simulink library "tp333079"  (Simulink 5.0)
values from neighbouring files (symbols this model uses):
  b = 1    [main_flock3.m]    (also in main_flock4.m; params_flocking_ros.m)
undefined symbols (not defined in the file or in its folder): AC, AlphaBnd, BetaBnd, CDda, CDde, CDdf, CDdr, CDM, CDmin, CGempty, CGgross, CL0, CLa, CLalphadot, Clbeta, Clda, CLde, CLdf, Cldr, CLM, CLmind, Clp, CLq, Clr, Cm0, Cma, Cmalphadot, Cmde, Cmdf, CmM, Cmq, Cnbeta, Cnda, Cndr, Cnp, Cnr, CP, CT, CYbeta, CYda, CYdr, CYp, CYr, Displacement, dmy, Engine, EulerIni, FuelFlow, FuelIni, J, Jempty, Jeng, Jgross, Jprop, MAC, MAP, MAPLim, MassIni, MaxPower, mempty ... (+26)
libraries: aerosimlib x325, simulink3 x42
(part 3 of 11)

== system tp333079/Atmosphere/Wind Shear ==
  note: Transversal wind shear
  note: Time derivatives of wind speed
      | in body axes
  note: Body velocities
  note: Lateral wind shear
  note: Vertical wind shear
  WindAcc : Inport  Port=1  PortDimensions=[3 1]  SampleTime=-1  DataType=auto
      settings: SignalType=auto
  TurbAcc : Inport  Port=2  PortDimensions=[3 1]  SampleTime=-1  DataType=auto
      settings: SignalType=auto
  Velocities : Inport  Port=3  PortDimensions=[3 1]  SampleTime=-1  DataType=auto
      settings: SignalType=auto
  Demux : Demux  Outputs=3  BusSelectionMode=off
  Demux1 : Demux  Outputs=3  BusSelectionMode=off
  Derivative : Derivative
  Mux : Mux  Inputs=3
  Mux1 : Mux  Inputs=3
  Product1 : Product  Inputs=*/  Multiplication=Element-wise(.*)  SaturateOnIntegerOverflow=on
  Product2 : Product  Inputs=*/  Multiplication=Element-wise(.*)  SaturateOnIntegerOverflow=on
  Product3 : Product  Inputs=*/  Multiplication=Element-wise(.*)  SaturateOnIntegerOverflow=on
  Sum : Sum  Inputs=|++  SaturateOnIntegerOverflow=on
  Terminator : Terminator
  Terminator1 : Terminator
  Terminator2 : Terminator
  Zero : Constant  Value=0
  Zero Offset : aerosimlib/Math/Zero Offset  tol=10^-6
  Zero Offset1 : Subsystem  SimViewingDevice=off  mask(Zero offset){tol=10^-6}
      mask prompts: tol "Tolerance"
      mask help: This block outputs a value equal to the tolerance specified in the block parameters if the input falls within a sphere with this tolerance as radius and center in the origin. Otherwise, the output equals the input.
      settings: Permissions=ReadWrite  RTWFcnNameOpts=Auto  RTWFileNameOpts=Auto
  Zero Offset2 : Subsystem  SimViewingDevice=off  mask(Zero offset){tol=10^-6}
      mask prompts: tol "Tolerance"
      mask help: This block outputs a value equal to the tolerance specified in the block parameters if the input falls within a sphere with this tolerance as radius and center in the origin. Otherwise, the output equals the input.
      settings: Permissions=ReadWrite  RTWFcnNameOpts=Auto  RTWFileNameOpts=Auto
  WindAngRates : Outport  Port=1
  WindAngAcc : Outport  Port=2
  wires:
  Product3/1 -> Terminator2/1
  Mux1/1 -> Derivative/1
  Zero Offset2/1(Out) -> Product1/2
  Zero Offset1/1(Out) -> Product2/2
  Derivative/1 -> WindAngAcc/1
  Sum/1 -> Demux1/1
  TurbAcc/1 -> Sum/2
  WindAcc/1 -> Sum/1
  Mux/1 -> WindAngRates/1
  Zero/1 -> Mux/1, Mux1/1, Mux1/3, Mux1/2
  Demux1/2 -> Product2/1
  Demux1/3 -> Product1/1, Product3/1
  Demux1/1 -> Terminator/1
  Velocities/1 -> Demux/1
  Demux/1 -> Zero Offset2/1(In), Zero Offset1/1(In)
  Demux/2 -> Zero Offset/1
  Demux/3 -> Terminator1/1
  Product1/1 -> Mux/2
  Product2/1 -> Mux/3
  Zero Offset/1 -> Product3/2

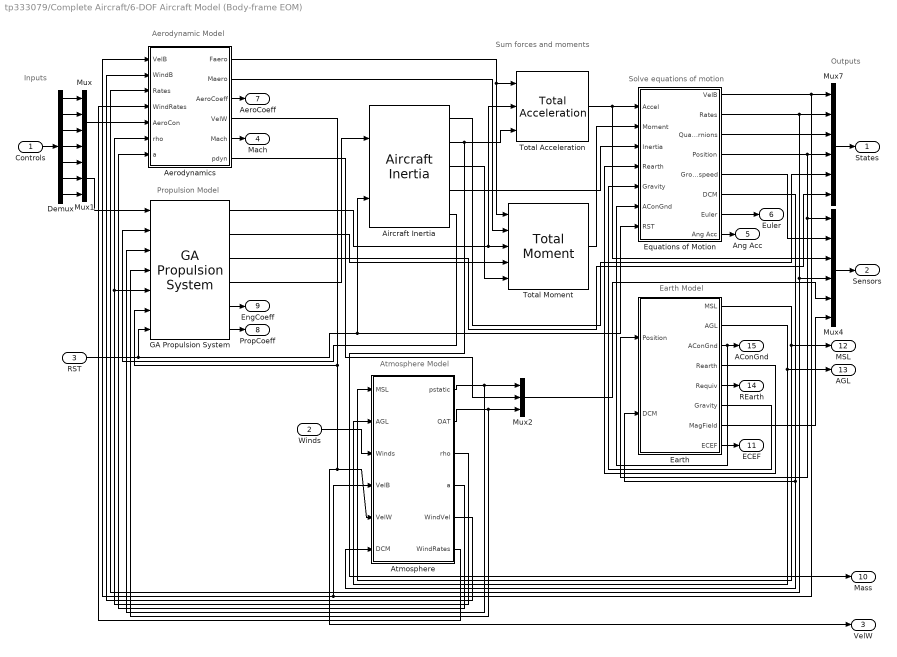
== system tp333079/Complete Aircraft/6-DOF Aircraft Model (Body-frame EOM) ==
  note: Propulsion Model
  note: Atmosphere Model
  note: Sum forces and moments
  note: Earth Model
  note: Aerodynamic Model
  note: Outputs
  note: Inputs
  note: Solve equations of motion
  Controls : Inport  Port=1  PortDimensions=-1  SampleTime=-1  DataType=auto
      settings: SignalType=auto
  Winds : Inport  Port=2  PortDimensions=-1  SampleTime=-1  DataType=auto
      settings: SignalType=auto
  RST : Inport  Port=3  PortDimensions=-1  SampleTime=-1  DataType=auto
      settings: SignalType=auto
  Aerodynamics : Subsystem  SimViewingDevice=off
      settings: Permissions=ReadWrite  RTWFcnNameOpts=Auto  RTWFileNameOpts=Auto
  Aircraft Inertia : aerosimlib/Inertia/Aircraft Inertia  FuelIni=FuelIni  Mempty=mempty  Mgross=mgross  CGempty=CGempty  CGgross=CGgross  Jempty=Jempty  Jgross=Jgross
  Atmosphere : Subsystem  SimViewingDevice=off
      settings: Permissions=ReadWrite  RTWFcnNameOpts=Auto  RTWFileNameOpts=Auto
  Demux : Demux  Outputs=7  BusSelectionMode=off
  Earth : Subsystem  SimViewingDevice=off
      settings: Permissions=ReadWrite  RTWFcnNameOpts=Auto  RTWFileNameOpts=Auto
  Equations of Motion : Subsystem  SimViewingDevice=off
      settings: Permissions=ReadWrite  RTWFcnNameOpts=Auto  RTWFileNameOpts=Auto
  GA Propulsion System : aerosimlib/Propulsion/GA Propulsion System  OmegaIni=OmegaIni  RPM=RPM  MAP=MAP  FuelFlow=FuelFlow  Power=Power  Jeng=Jeng  J=J  CT=CT  CP=CP  Rprop=Rprop  Jprop=Jprop  TSL=TSL
  Mux : Mux  Inputs=4
  Mux1 : Mux  Inputs=3
  Mux2 : Mux  Inputs=3
  Mux4 : Mux  Inputs=6
  Mux7 : Mux  Inputs=6
  Total Acceleration : aerosimlib/Equations of Motion/Total Acceleration
  Total Moment : aerosimlib/Equations of Motion/Total Moment  raero=rAC  rprop=rHub
  States : Outport  Port=1
  Sensors : Outport  Port=2
  VelW : Outport  Port=3
  Mach : Outport  Port=4
  Ang Acc : Outport  Port=5
  Euler : Outport  Port=6
  AeroCoeff : Outport  Port=7
  PropCoeff : Outport  Port=8
  EngCoeff : Outport  Port=9
  Mass : Outport  Port=10
  ECEF : Outport  Port=11
  MSL : Outport  Port=12
  AGL : Outport  Port=13
  REarth : Outport  Port=14
  AConGnd : Outport  Port=15
  wires:
  Earth/8(ECEF) -> ECEF/1
  Aerodynamics/3(AeroCoeff) -> AeroCoeff/1
  Aerodynamics/5(Mach) -> Mach/1
  Equations of Motion/3(Quaternions) -> Mux7/3
  Mux/1 -> Aerodynamics/5(AeroCon)
  Equations of Motion/4(Position) -> Mux7/4, Mux4/1, Earth/1(Position)
  Equations of Motion/2(Rates) -> Mux7/2, Mux4/4, Aerodynamics/3(Rates)
  Equations of Motion/1(VelB) -> Mux7/1, Atmosphere/4(VelB), Aerodynamics/1(VelB)
  Mux1/1 -> GA Propulsion System/1
  Mux7/1 -> States/1
  Mux4/1 -> Sensors/1
  Controls/1 -> Demux/1
  Demux/1 -> Mux/1
  Demux/2 -> Mux/2
  Demux/3 -> Mux/3
  Demux/4 -> Mux/4
  Demux/5 -> Mux1/1
  Demux/6 -> Mux1/2
  Demux/7 -> Mux1/3
  GA Propulsion System/5 -> EngCoeff/1
  GA Propulsion System/6 -> PropCoeff/1
  Earth/5(Requiv) -> REarth/1
  Earth/3(AConGnd) -> AConGnd/1, Equations of Motion/6(AConGnd)
  Equations of Motion/5(Groundspeed) -> Mux4/2
  Total Acceleration/1 -> Equations of Motion/1(Accel), Mux4/3
  Earth/7(MagField) -> Mux4/6
  Earth/6(Gravity) -> Equations of Motion/5(Gravity)
  Earth/4(Rearth) -> Equations of Motion/4(Rearth)
  Aircraft Inertia/2 -> Total Acceleration/3, Mass/1
  Aircraft Inertia/4 -> Equations of Motion/3(Inertia)
  Total Moment/1 -> Equations of Motion/2(Moment)
  Aircraft Inertia/3 -> Total Moment/5
  Aerodynamics/1(Faero) -> Total Acceleration/1, Total Moment/1
  Aerodynamics/2(Maero) -> Total Moment/2
  GA Propulsion System/1 -> Total Acceleration/2, Total Moment/3
  GA Propulsion System/2 -> Total Moment/4
  Equations of Motion/6(DCM) -> Earth/2(DCM), Atmosphere/6(DCM)
  Atmosphere/1(pstatic) -> Mux2/1, GA Propulsion System/3
  Atmosphere/2(OAT) -> Mux2/3, GA Propulsion System/4
  Aerodynamics/6(pdyn) -> Mux2/2
  Mux2/1 -> Mux4/5
  Aircraft Inertia/1 -> Mux7/5
  GA Propulsion System/3 -> Mux7/6
  GA Propulsion System/4 -> Aircraft Inertia/1
  Aerodynamics/4(VelW) -> GA Propulsion System/6, Atmosphere/5(VelW), VelW/1
  Earth/1(MSL) -> Atmosphere/1(MSL), MSL/1
  Earth/2(AGL) -> Atmosphere/2(AGL), AGL/1
  Winds/1 -> Atmosphere/3(Winds)
  Atmosphere/5(WindVel) -> Aerodynamics/2(WindB)
  Atmosphere/3(rho) -> Aerodynamics/6(rho), GA Propulsion System/5
  Atmosphere/4(a) -> Aerodynamics/7(a)
  Aircraft Inertia/5 -> GA Propulsion System/2
  RST/1 -> GA Propulsion System/7, Equations of Motion/7(RST), Aircraft Inertia/2
  Atmosphere/6(WindRates) -> Aerodynamics/4(WindRates)
  Equations of Motion/8(Ang Acc) -> Ang Acc/1
  Equations of Motion/7(Euler) -> Euler/1

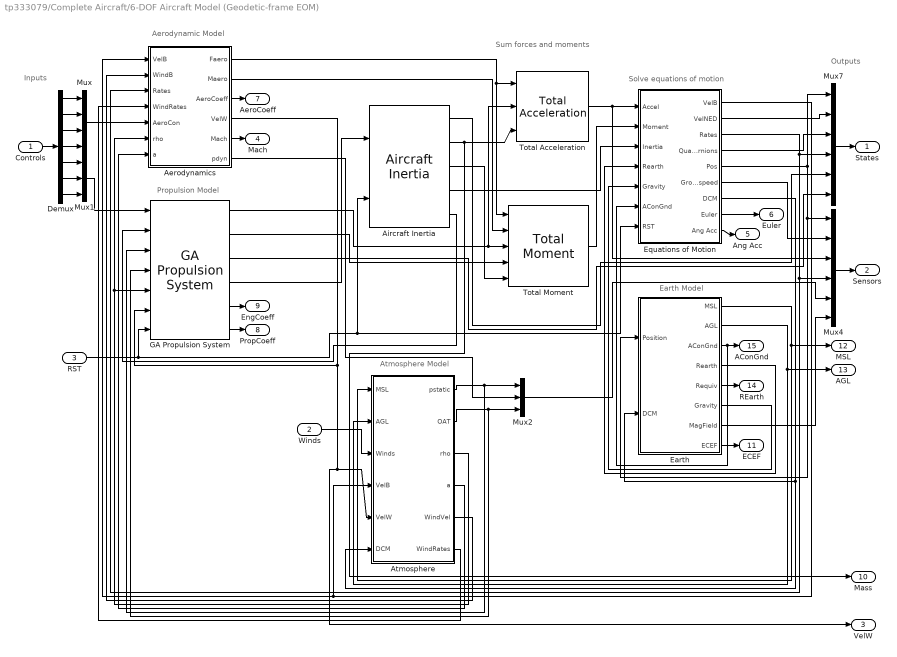
== system tp333079/Complete Aircraft/6-DOF Aircraft Model (Geodetic-frame EOM) ==
  note: Propulsion Model
  note: Atmosphere Model
  note: Sum forces and moments
  note: Earth Model
  note: Aerodynamic Model
  note: Outputs
  note: Inputs
  note: Solve equations of motion
  Controls : Inport  Port=1  PortDimensions=-1  SampleTime=-1  DataType=auto
      settings: SignalType=auto
  Winds : Inport  Port=2  PortDimensions=-1  SampleTime=-1  DataType=auto
      settings: SignalType=auto
  RST : Inport  Port=3  PortDimensions=-1  SampleTime=-1  DataType=auto
      settings: SignalType=auto
  Aerodynamics : Subsystem  SimViewingDevice=off
      settings: Permissions=ReadWrite  RTWFcnNameOpts=Auto  RTWFileNameOpts=Auto
  Aircraft Inertia : aerosimlib/Inertia/Aircraft Inertia  FuelIni=FuelIni  Mempty=mempty  Mgross=mgross  CGempty=CGempty  CGgross=CGgross  Jempty=Jempty  Jgross=Jgross
  Atmosphere : Subsystem  SimViewingDevice=off
      settings: Permissions=ReadWrite  RTWFcnNameOpts=Auto  RTWFileNameOpts=Auto
  Demux : Demux  Outputs=7  BusSelectionMode=off
  Earth : Subsystem  SimViewingDevice=off
      settings: Permissions=ReadWrite  RTWFcnNameOpts=Auto  RTWFileNameOpts=Auto
  Equations of Motion : Subsystem  SimViewingDevice=off
      settings: Permissions=ReadWrite  RTWFcnNameOpts=Auto  RTWFileNameOpts=Auto
  GA Propulsion System : aerosimlib/Propulsion/GA Propulsion System  OmegaIni=OmegaIni  RPM=RPM  MAP=MAP  FuelFlow=FuelFlow  Power=Power  Jeng=Jeng  J=J  CT=CT  CP=CP  Rprop=Rprop  Jprop=Jprop  TSL=TSL
  Mux : Mux  Inputs=4
  Mux1 : Mux  Inputs=3
  Mux2 : Mux  Inputs=3
  Mux4 : Mux  Inputs=6
  Mux7 : Mux  Inputs=6
  Total Acceleration : aerosimlib/Equations of Motion/Total Acceleration
  Total Moment : aerosimlib/Equations of Motion/Total Moment  raero=rAC  rprop=rHub
  States : Outport  Port=1
  Sensors : Outport  Port=2
  VelW : Outport  Port=3
  Mach : Outport  Port=4
  Ang Acc : Outport  Port=5
  Euler : Outport  Port=6
  AeroCoeff : Outport  Port=7
  PropCoeff : Outport  Port=8
  EngCoeff : Outport  Port=9
  Mass : Outport  Port=10
  ECEF : Outport  Port=11
  MSL : Outport  Port=12
  AGL : Outport  Port=13
  REarth : Outport  Port=14
  AConGnd : Outport  Port=15
  wires:
  Earth/8(ECEF) -> ECEF/1
  Aerodynamics/3(AeroCoeff) -> AeroCoeff/1
  Aerodynamics/5(Mach) -> Mach/1
  Mux/1 -> Aerodynamics/5(AeroCon)
  Equations of Motion/5(Pos) -> Mux4/1, Earth/1(Position), Mux7/1
  Equations of Motion/3(Rates) -> Mux4/4, Aerodynamics/3(Rates), Mux7/4
  Equations of Motion/1(VelB) -> Atmosphere/4(VelB), Aerodynamics/1(VelB)
  Mux1/1 -> GA Propulsion System/1
  Mux7/1 -> States/1
  Mux4/1 -> Sensors/1
  Controls/1 -> Demux/1
  Demux/1 -> Mux/1
  Demux/2 -> Mux/2
  Demux/3 -> Mux/3
  Demux/4 -> Mux/4
  Demux/5 -> Mux1/1
  Demux/6 -> Mux1/2
  Demux/7 -> Mux1/3
  GA Propulsion System/5 -> EngCoeff/1
  GA Propulsion System/6 -> PropCoeff/1
  Earth/5(Requiv) -> REarth/1
  Earth/3(AConGnd) -> AConGnd/1, Equations of Motion/6(AConGnd)
  Equations of Motion/6(Groundspeed) -> Mux4/2
  Total Acceleration/1 -> Equations of Motion/1(Accel), Mux4/3
  Earth/7(MagField) -> Mux4/6
  Earth/6(Gravity) -> Equations of Motion/5(Gravity)
  Earth/4(Rearth) -> Equations of Motion/4(Rearth)
  Aircraft Inertia/2 -> Total Acceleration/3, Mass/1
  Aircraft Inertia/4 -> Equations of Motion/3(Inertia)
  Total Moment/1 -> Equations of Motion/2(Moment)
  Aircraft Inertia/3 -> Total Moment/5
  Aerodynamics/1(Faero) -> Total Acceleration/1, Total Moment/1
  Aerodynamics/2(Maero) -> Total Moment/2
  GA Propulsion System/1 -> Total Acceleration/2, Total Moment/3
  GA Propulsion System/2 -> Total Moment/4
  Equations of Motion/7(DCM) -> Earth/2(DCM), Atmosphere/6(DCM)
  Atmosphere/1(pstatic) -> Mux2/1, GA Propulsion System/3
  Atmosphere/2(OAT) -> Mux2/3, GA Propulsion System/4
  Aerodynamics/6(pdyn) -> Mux2/2
  Mux2/1 -> Mux4/5
  Aircraft Inertia/1 -> Mux7/5
  GA Propulsion System/3 -> Mux7/6
  GA Propulsion System/4 -> Aircraft Inertia/1
  Aerodynamics/4(VelW) -> GA Propulsion System/6, Atmosphere/5(VelW), VelW/1
  Earth/1(MSL) -> Atmosphere/1(MSL), MSL/1
  Earth/2(AGL) -> Atmosphere/2(AGL), AGL/1
  Winds/1 -> Atmosphere/3(Winds)
  Atmosphere/5(WindVel) -> Aerodynamics/2(WindB)
  Atmosphere/3(rho) -> Aerodynamics/6(rho), GA Propulsion System/5
  Atmosphere/4(a) -> Aerodynamics/7(a)
  Aircraft Inertia/5 -> GA Propulsion System/2
  RST/1 -> GA Propulsion System/7, Equations of Motion/7(RST), Aircraft Inertia/2
  Atmosphere/6(WindRates) -> Aerodynamics/4(WindRates)
  Equations of Motion/9(Ang Acc) -> Ang Acc/1
  Equations of Motion/8(Euler) -> Euler/1
  Equations of Motion/2(VelNED) -> Mux7/2
  Equations of Motion/4(Quaternions) -> Mux7/3

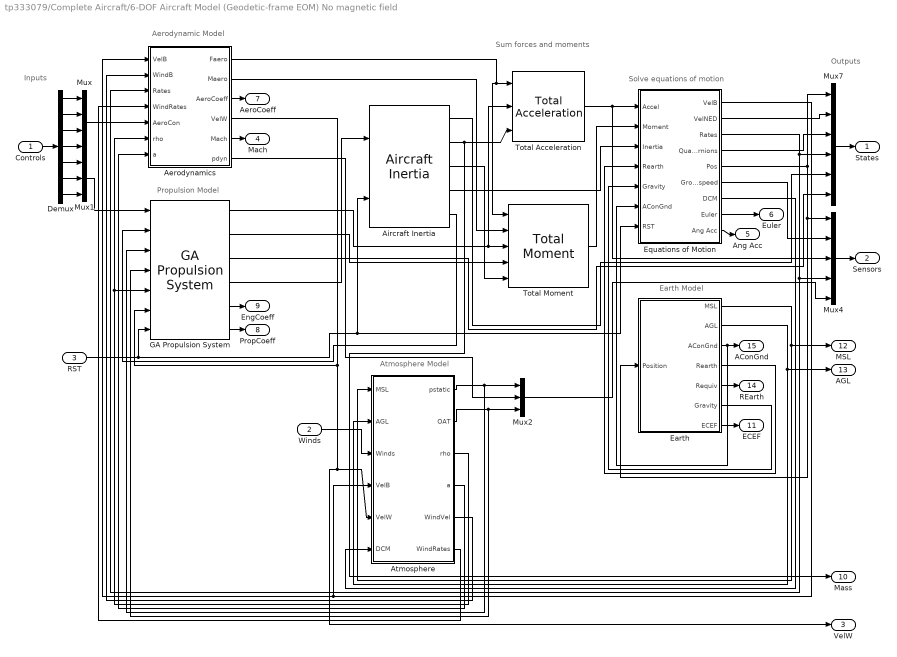
== system tp333079/Complete Aircraft/6-DOF Aircraft Model (Geodetic-frame EOM) No magnetic field ==
  note: Solve equations of motion
  note: Inputs
  note: Outputs
  note: Aerodynamic Model
  note: Earth Model
  note: Sum forces and moments
  note: Atmosphere Model
  note: Propulsion Model
  Controls : Inport  Port=1  PortDimensions=-1  SampleTime=-1  DataType=auto
      settings: SignalType=auto
  Winds : Inport  Port=2  PortDimensions=-1  SampleTime=-1  DataType=auto
      settings: SignalType=auto
  RST : Inport  Port=3  PortDimensions=-1  SampleTime=-1  DataType=auto
      settings: SignalType=auto
  Aerodynamics : Subsystem  SimViewingDevice=off
      settings: Permissions=ReadWrite  RTWFcnNameOpts=Auto  RTWFileNameOpts=Auto
  Aircraft Inertia : aerosimlib/Inertia/Aircraft Inertia  FuelIni=FuelIni  Mempty=mempty  Mgross=mgross  CGempty=CGempty  CGgross=CGgross  Jempty=Jempty  Jgross=Jgross
  Atmosphere : Subsystem  SimViewingDevice=off
      settings: Permissions=ReadWrite  RTWFcnNameOpts=Auto  RTWFileNameOpts=Auto
  Demux : Demux  Outputs=7  BusSelectionMode=off
  Earth : Subsystem  SimViewingDevice=off
      settings: Permissions=ReadWrite  RTWFcnNameOpts=Auto  RTWFileNameOpts=Auto
  Equations of Motion : Subsystem  SimViewingDevice=off
      settings: Permissions=ReadWrite  RTWFcnNameOpts=Auto  RTWFileNameOpts=Auto
  GA Propulsion System : aerosimlib/Propulsion/GA Propulsion System  OmegaIni=OmegaIni  RPM=RPM  MAP=MAP  FuelFlow=FuelFlow  Power=Power  Jeng=Jeng  J=J  CT=CT  CP=CP  Rprop=Rprop  Jprop=Jprop  TSL=TSL
  Mux : Mux  Inputs=4
  Mux1 : Mux  Inputs=3
  Mux2 : Mux  Inputs=3
  Mux4 : Mux  Inputs=5
  Mux7 : Mux  Inputs=6
  Total Acceleration : aerosimlib/Equations of Motion/Total Acceleration
  Total Moment : aerosimlib/Equations of Motion/Total Moment  raero=rAC  rprop=rHub
  States : Outport  Port=1
  Sensors : Outport  Port=2
  VelW : Outport  Port=3
  Mach : Outport  Port=4
  Ang Acc : Outport  Port=5
  Euler : Outport  Port=6
  AeroCoeff : Outport  Port=7
  PropCoeff : Outport  Port=8
  EngCoeff : Outport  Port=9
  Mass : Outport  Port=10
  ECEF : Outport  Port=11
  MSL : Outport  Port=12
  AGL : Outport  Port=13
  REarth : Outport  Port=14
  AConGnd : Outport  Port=15
  wires:
  Equations of Motion/4(Quaternions) -> Mux7/3
  Equations of Motion/2(VelNED) -> Mux7/2
  Equations of Motion/8(Euler) -> Euler/1
  Equations of Motion/9(Ang Acc) -> Ang Acc/1
  Atmosphere/6(WindRates) -> Aerodynamics/4(WindRates)
  RST/1 -> Aircraft Inertia/2, Equations of Motion/7(RST), GA Propulsion System/7
  Aircraft Inertia/5 -> GA Propulsion System/2
  Atmosphere/4(a) -> Aerodynamics/7(a)
  Atmosphere/3(rho) -> GA Propulsion System/5, Aerodynamics/6(rho)
  Atmosphere/5(WindVel) -> Aerodynamics/2(WindB)
  Winds/1 -> Atmosphere/3(Winds)
  Earth/2(AGL) -> AGL/1, Atmosphere/2(AGL)
  Earth/1(MSL) -> MSL/1, Atmosphere/1(MSL)
  Aerodynamics/4(VelW) -> VelW/1, Atmosphere/5(VelW), GA Propulsion System/6
  GA Propulsion System/4 -> Aircraft Inertia/1
  GA Propulsion System/3 -> Mux7/6
  Aircraft Inertia/1 -> Mux7/5
  Mux2/1 -> Mux4/5
  Aerodynamics/6(pdyn) -> Mux2/2
  Atmosphere/2(OAT) -> GA Propulsion System/4, Mux2/3
  Atmosphere/1(pstatic) -> GA Propulsion System/3, Mux2/1
  Equations of Motion/7(DCM) -> Atmosphere/6(DCM)
  GA Propulsion System/2 -> Total Moment/4
  GA Propulsion System/1 -> Total Acceleration/2, Total Moment/3
  Aerodynamics/1(Faero) -> Total Acceleration/1, Total Moment/1
  Aircraft Inertia/3 -> Total Moment/5
  Total Moment/1 -> Equations of Motion/2(Moment)
  Aircraft Inertia/4 -> Equations of Motion/3(Inertia)
  Aircraft Inertia/2 -> Total Acceleration/3, Mass/1
  Earth/4(Rearth) -> Equations of Motion/4(Rearth)
  Earth/6(Gravity) -> Equations of Motion/5(Gravity)
  Total Acceleration/1 -> Mux4/3, Equations of Motion/1(Accel)
  Equations of Motion/6(Groundspeed) -> Mux4/2
  Earth/3(AConGnd) -> Equations of Motion/6(AConGnd), AConGnd/1
  Earth/5(Requiv) -> REarth/1
  GA Propulsion System/6 -> PropCoeff/1
  GA Propulsion System/5 -> EngCoeff/1
  Demux/7 -> Mux1/3
  Demux/6 -> Mux1/2
  Demux/5 -> Mux1/1
  Demux/4 -> Mux/4
  Demux/3 -> Mux/3
  Demux/2 -> Mux/2
  Demux/1 -> Mux/1
  Controls/1 -> Demux/1
  Mux4/1 -> Sensors/1
  Mux7/1 -> States/1
  Mux1/1 -> GA Propulsion System/1
  Equations of Motion/1(VelB) -> Aerodynamics/1(VelB), Atmosphere/4(VelB)
  Equations of Motion/3(Rates) -> Mux7/4, Mux4/4, Aerodynamics/3(Rates)
  Equations of Motion/5(Pos) -> Mux7/1, Earth/1(Position), Mux4/1
  Mux/1 -> Aerodynamics/5(AeroCon)
  Aerodynamics/5(Mach) -> Mach/1
  Aerodynamics/3(AeroCoeff) -> AeroCoeff/1
  Earth/7(ECEF) -> ECEF/1
  Aerodynamics/2(Maero) -> Total Moment/2

== system tp333079/Complete Aircraft/Glider Model ==
  note: Sum forces and moments
  note: Aerodynamic Model
  note: Outputs
  note: Inputs
  note: Solve equations of motion
  Controls : Inport  Port=1  PortDimensions=-1  SampleTime=-1  DataType=auto
      settings: SignalType=auto
  Aerodynamics : aerosimlib/Complete Aircraft/6-DOF Aircraft Model (Body-frame EOM)/Aerodynamics  SimViewingDevice=off
      settings: Permissions=ReadWrite  RTWFcnNameOpts=Auto  RTWFileNameOpts=Auto
  Aircraft Inertia : aerosimlib/Inertia/Aircraft Inertia  FuelIni=0  Mempty=mempty  Mgross=mgross  CGempty=CGempty  CGgross=CGgross  Jempty=Jempty  Jgross=Jgross
  Constant{,5,7..8} (4 alike) : Constant  Value=0
  Constant3 : Constant  Value=zeros(3,1)
  Constant4 : Constant  Value=zeros(3,1)
  Demux1 : Demux  Outputs=3  BusSelectionMode=off
  Equations of Motion : Subsystem  SimViewingDevice=off
      settings: Permissions=ReadWrite  RTWFcnNameOpts=Auto  RTWFileNameOpts=Auto
  Mux2 : Mux  Inputs=3
  Mux3 : Mux  Orientation=left  Inputs=2
  Mux4 : Mux  Inputs=5
  Mux7 : Mux  Inputs=4
  Standard Atmosphere : aerosimlib/Atmosphere/Standard Atmosphere
  Terminator{1..6} (6 alike) : Terminator
  Total Acceleration : aerosimlib/Equations of Motion/Total Acceleration
  Total Moment : aerosimlib/Equations of Motion/Total Moment  raero=rAC  rprop=rHub
  WGS-84 : aerosimlib/Earth/WGS-84  Orientation=left
  States : Outport  Port=1
  Sensors : Outport  Port=2
  VelW : Outport  Port=3
  Mach : Outport  Port=4
  Ang Acc : Outport  Port=5
  Euler : Outport  Port=6
  AeroCoeff : Outport  Port=7
  wires:
  Aerodynamics/3 -> AeroCoeff/1
  Aerodynamics/5 -> Mach/1
  Equations of Motion/3(Quaternions) -> Mux7/3
  Equations of Motion/4(Position) -> Mux7/4, Mux4/1, Demux1/1, WGS-84/1
  Equations of Motion/2(Rates) -> Mux7/2, Mux4/4, Aerodynamics/3
  Equations of Motion/1(VelB) -> Mux7/1, Aerodynamics/1
  Mux7/1 -> States/1
  Mux4/1 -> Sensors/1
  Controls/1 -> Aerodynamics/5
  Equations of Motion/5(Groundspeed) -> Mux4/2
  Total Acceleration/1 -> Equations of Motion/1(Accel), Mux4/3
  Aircraft Inertia/2 -> Total Acceleration/3
  Aircraft Inertia/4 -> Equations of Motion/3(Inertia)
  Total Moment/1 -> Equations of Motion/2(Moment)
  Aircraft Inertia/3 -> Total Moment/5
  Aerodynamics/1 -> Total Acceleration/1, Total Moment/1
  Aerodynamics/2 -> Total Moment/2
  Aerodynamics/6 -> Mux2/2
  Mux2/1 -> Mux4/5
  Aerodynamics/4 -> VelW/1
  Equations of Motion/7(Euler) -> Euler/1
  Equations of Motion/8(Ang Acc) -> Ang Acc/1
  Constant/1 -> Equations of Motion/6(AConGnd)
  Constant7/1 -> Equations of Motion/7(RST)
  Equations of Motion/6(DCM) -> Terminator2/1
  Demux1/1 -> Terminator1/1
  Demux1/2 -> Terminator3/1
  Demux1/3 -> Standard Atmosphere/1
  Standard Atmosphere/1 -> Mux2/1
  Standard Atmosphere/2 -> Mux2/3
  Standard Atmosphere/3 -> Aerodynamics/6
  Standard Atmosphere/4 -> Aerodynamics/7
  Constant3/1 -> Aerodynamics/2
  Constant4/1 -> Aerodynamics/4
  Constant8/1 -> Aircraft Inertia/2
  Constant5/1 -> Aircraft Inertia/1
  Aircraft Inertia/5 -> Terminator4/1
  Aircraft Inertia/1 -> Terminator5/1
  WGS-84/1 -> Mux3/1
  WGS-84/2 -> Mux3/2
  WGS-84/3 -> Terminator6/1
  Mux3/1 -> Equations of Motion/4(Rearth)
  WGS-84/4 -> Equations of Motion/5(Gravity)

== system tp333079/Complete Aircraft/Inertial Navigation System ==
  IMU : Inport  Port=1  PortDimensions=[6 1]  SampleTime=tsamp  DataType=auto
      settings: SignalType=auto
  RST : Inport  Port=2  PortDimensions=1  SampleTime=tsamp  DataType=auto
      settings: SignalType=auto
  Attitude : aerosimlib/Equations of Motion/Body-Frame EOM/Kinematics (Quaternions)  QuaternionsIni=QuaternionsIni
  Body-Inertial DCM : aerosimlib/Transformations/Body-Inertial DCM From Quaternions  Orientation=left
  Constant : Constant  Value=0
  Demux : Demux  Outputs=2  BusSelectionMode=off
  Mux : Mux  Inputs=3
  Position : aerosimlib/Equations of Motion/Geodetic-Frame EOM/Position  PositionIni=PositionIni
  Terminator : Terminator
  Velocity : aerosimlib/Equations of Motion/Geodetic-Frame EOM/Velocity  VelocitiesIni=VelocitiesIni
  WGS-84 : aerosimlib/Earth/WGS-84
  PVA : Outport  Port=1
  wires:
  IMU/1 -> Demux/1
  WGS-84/3 -> Terminator/1
  Velocity/1 -> Position/1, Mux/2
  WGS-84/1 -> Position/2
  WGS-84/2 -> Position/3
  WGS-84/4 -> Velocity/5
  Demux/1 -> Velocity/3
  Demux/2 -> Attitude/1
  RST/1 -> Attitude/2, Position/5, Velocity/6
  Attitude/1 -> Mux/3, Body-Inertial DCM/1
  Position/1 -> Velocity/1, WGS-84/1, Mux/1
  Position/2 -> Velocity/2
  Constant/1 -> Position/4
  Mux/1 -> PVA/1
  Body-Inertial DCM/1 -> Velocity/4

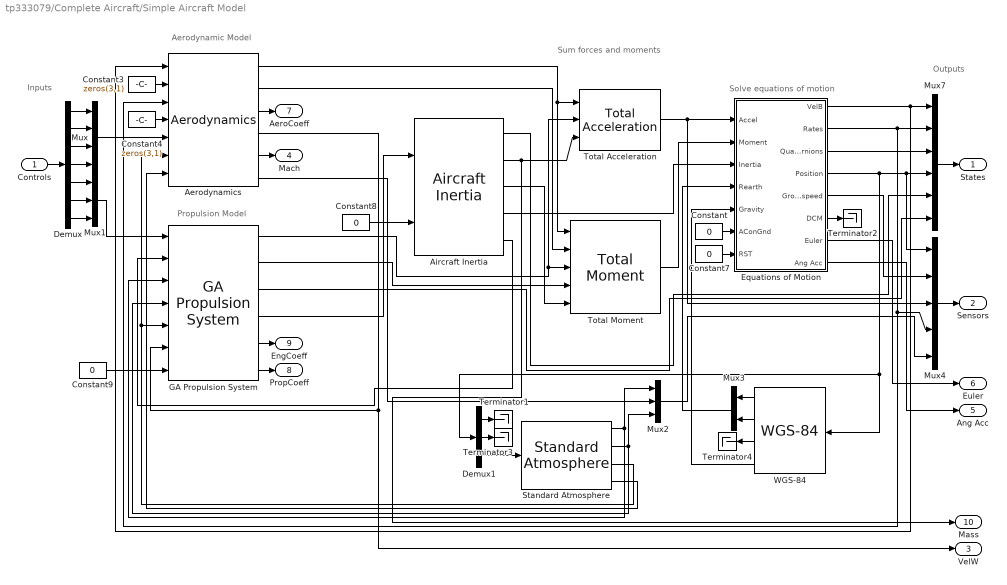
== system tp333079/Complete Aircraft/Simple Aircraft Model ==
  note: Propulsion Model
  note: Sum forces and moments
  note: Aerodynamic Model
  note: Outputs
  note: Inputs
  note: Solve equations of motion
  Controls : Inport  Port=1  PortDimensions=-1  SampleTime=-1  DataType=auto
      settings: SignalType=auto
  Aerodynamics : aerosimlib/Complete Aircraft/6-DOF Aircraft Model (Body-frame EOM)/Aerodynamics  SimViewingDevice=off
      settings: Permissions=ReadWrite  RTWFcnNameOpts=Auto  RTWFileNameOpts=Auto
  Aircraft Inertia : aerosimlib/Inertia/Aircraft Inertia  FuelIni=FuelIni  Mempty=mempty  Mgross=mgross  CGempty=CGempty  CGgross=CGgross  Jempty=Jempty  Jgross=Jgross
  Constant{,7..9} (4 alike) : Constant  Value=0
  Constant3 : Constant  Value=zeros(3,1)
  Constant4 : Constant  Value=zeros(3,1)
  Demux : Demux  Outputs=7  BusSelectionMode=off
  Demux1 : Demux  Outputs=3  BusSelectionMode=off
  Equations of Motion : Subsystem  SimViewingDevice=off
      settings: Permissions=ReadWrite  RTWFcnNameOpts=Auto  RTWFileNameOpts=Auto
  GA Propulsion System : aerosimlib/Propulsion/GA Propulsion System  OmegaIni=OmegaIni  RPM=RPM  MAP=MAP  FuelFlow=FuelFlow  Power=Power  Jeng=Jeng  J=J  CT=CT  CP=CP  Rprop=Rprop  Jprop=Jprop  TSL=TSL
  Mux : Mux  Inputs=4
  Mux1 : Mux  Inputs=3
  Mux2 : Mux  Inputs=3
  Mux3 : Mux  Orientation=left  Inputs=2
  Mux4 : Mux  Inputs=5
  Mux7 : Mux  Inputs=6
  Standard Atmosphere : aerosimlib/Atmosphere/Standard Atmosphere
  Terminator{1..4} (4 alike) : Terminator
  Total Acceleration : aerosimlib/Equations of Motion/Total Acceleration
  Total Moment : aerosimlib/Equations of Motion/Total Moment  raero=rAC  rprop=rHub
  WGS-84 : aerosimlib/Earth/WGS-84  Orientation=left
  States : Outport  Port=1
  Sensors : Outport  Port=2
  VelW : Outport  Port=3
  Mach : Outport  Port=4
  Ang Acc : Outport  Port=5
  Euler : Outport  Port=6
  AeroCoeff : Outport  Port=7
  PropCoeff : Outport  Port=8
  EngCoeff : Outport  Port=9
  Mass : Outport  Port=10
  wires:
  Aerodynamics/3 -> AeroCoeff/1
  Aerodynamics/5 -> Mach/1
  Equations of Motion/3(Quaternions) -> Mux7/3
  Mux/1 -> Aerodynamics/5
  Equations of Motion/4(Position) -> Mux7/4, Mux4/1, Demux1/1, WGS-84/1
  Equations of Motion/2(Rates) -> Mux7/2, Mux4/4, Aerodynamics/3
  Equations of Motion/1(VelB) -> Mux7/1, Aerodynamics/1
  Mux1/1 -> GA Propulsion System/1
  Mux7/1 -> States/1
  Mux4/1 -> Sensors/1
  Controls/1 -> Demux/1
  Demux/1 -> Mux/1
  Demux/2 -> Mux/2
  Demux/3 -> Mux/3
  Demux/4 -> Mux/4
  Demux/5 -> Mux1/1
  Demux/6 -> Mux1/2
  Demux/7 -> Mux1/3
  GA Propulsion System/5 -> EngCoeff/1
  GA Propulsion System/6 -> PropCoeff/1
  Equations of Motion/5(Groundspeed) -> Mux4/2
  Total Acceleration/1 -> Equations of Motion/1(Accel), Mux4/3
  Aircraft Inertia/2 -> Mass/1, Total Acceleration/3
  Aircraft Inertia/4 -> Equations of Motion/3(Inertia)
  Total Moment/1 -> Equations of Motion/2(Moment)
  Aircraft Inertia/3 -> Total Moment/5
  Aerodynamics/1 -> Total Acceleration/1, Total Moment/1
  GA Propulsion System/1 -> Total Acceleration/2, Total Moment/3
  GA Propulsion System/2 -> Total Moment/4
  Aerodynamics/6 -> Mux2/2
  Mux2/1 -> Mux4/5
  Aircraft Inertia/1 -> Mux7/5
  GA Propulsion System/3 -> Mux7/6
  GA Propulsion System/4 -> Aircraft Inertia/1
  Aerodynamics/4 -> GA Propulsion System/6, VelW/1
  Aircraft Inertia/5 -> GA Propulsion System/2
  Equations of Motion/7(Euler) -> Euler/1
  Equations of Motion/8(Ang Acc) -> Ang Acc/1
  Constant/1 -> Equations of Motion/6(AConGnd)
  Constant7/1 -> Equations of Motion/7(RST)
  Equations of Motion/6(DCM) -> Terminator2/1
  Demux1/1 -> Terminator1/1
  Demux1/2 -> Terminator3/1
  Demux1/3 -> Standard Atmosphere/1
  Standard Atmosphere/1 -> Mux2/1, GA Propulsion System/3
  Standard Atmosphere/2 -> Mux2/3, GA Propulsion System/4
  Standard Atmosphere/3 -> Aerodynamics/6, GA Propulsion System/5
  Standard Atmosphere/4 -> Aerodynamics/7
  Constant3/1 -> Aerodynamics/2
  Constant4/1 -> Aerodynamics/4
  Constant8/1 -> Aircraft Inertia/2
  Constant9/1 -> GA Propulsion System/7
  Aerodynamics/2 -> Total Moment/2
  WGS-84/1 -> Mux3/1
  WGS-84/2 -> Mux3/2
  Mux3/1 -> Equations of Motion/4(Rearth)
  WGS-84/4 -> Equations of Motion/5(Gravity)
  WGS-84/3 -> Terminator4/1

== system tp333079/Earth/EGM-96 ==
  note: Sources
  note: Compute Mean-Sea Level Altitude
  Position : Inport  Port=1  PortDimensions=-1  SampleTime=-1  DataType=auto
      settings: SignalType=auto
  Demux2 : Demux  Outputs=3  BusSelectionMode=off
  Longitude Bound 0-2pi : Subsystem  SimViewingDevice=off
      settings: Permissions=ReadWrite  RTWFcnNameOpts=Auto  RTWFileNameOpts=Auto
      mask Type: Longitude bound
      mask Description: Bounds the longitude to [0, 2pi]. When 0 bound is exceeded the longitude wraps back to 2pi; when the 2pi bound is exceeded the longitude wraps back to 0.
  Look-Up Table (2-D) : simulink3/Functions & Tables/Look-Up Table (2-D)  x=Lat  y=Lon  t=Alterr'
  Sum : Sum  Inputs=+++  SaturateOnIntegerOverflow=on
  WGS-84 correction : Constant  Value=-0.53
  rad 2 deg : Subsystem  SimViewingDevice=off
      settings: Permissions=ReadWrite  RTWFcnNameOpts=Auto  RTWFileNameOpts=Auto
      mask Type: Radians to degrees
      mask Description: Convert radians to degrees.
      mask Display: disp('RAD DEG');
  rad 2 deg1 : Subsystem  SimViewingDevice=off
      settings: Permissions=ReadWrite  RTWFcnNameOpts=Auto  RTWFileNameOpts=Auto
      mask Type: Radians to degrees
      mask Description: Convert radians to degrees.
      mask Display: disp('RAD DEG');
  MSLAlt : Outport  Port=1
  wires:
  Longitude Bound 0-2pi/1(Out) -> rad 2 deg1/1(In)
  Position/1 -> Demux2/1
  Demux2/3 -> Sum/1
  Demux2/1 -> rad 2 deg/1(In)
  Demux2/2 -> Longitude Bound 0-2pi/1(In)
  rad 2 deg/1(Out) -> Look-Up Table (2-D)/1
  rad 2 deg1/1(Out) -> Look-Up Table (2-D)/2
  Look-Up Table (2-D)/1 -> Sum/2
  WGS-84 correction/1 -> Sum/3
  Sum/1 -> MSLAlt/1

== system tp333079/Earth/Ground Detection ==
  MSLAlt : Inport  Port=1  PortDimensions=-1  SampleTime=-1  DataType=auto
      settings: SignalType=auto
  GndAlt : Inport  Port=2  PortDimensions=-1  SampleTime=-1  DataType=auto
      settings: SignalType=auto
  False : Constant  Value=0
  Sum : Sum  Inputs=|+-  SaturateOnIntegerOverflow=on
  Switch : Switch  Threshold=0
  True : Constant  Value=1
  AConGnd : Outport  Port=1
  AGLAlt : Outport  Port=2
  wires:
  MSLAlt/1 -> Sum/1
  GndAlt/1 -> Sum/2
  Sum/1 -> Switch/2, AGLAlt/1
  False/1 -> Switch/1
  True/1 -> Switch/3
  Switch/1 -> AConGnd/1

== system tp333079/Earth/WGS-84 ==
  note: Sources
  note: Compute radii and surface gravity
  note: Correct gravity for altitude
  note: Outputs
  Position : Inport  Port=1  PortDimensions=-1  SampleTime=-1  DataType=auto
      settings: SignalType=auto
  1/2 : Constant  Value=1/2
  3/2 : Constant  Value=3/2
  Demux2 : Demux  Outputs=3  BusSelectionMode=off
  Equatorial Radius : Constant  Value=6378137
  First Eccentricity : Constant  Value=0.0818191908426
  Gravity at Equator : Constant  Value=9.7803267714
  Gravity formula const : Constant  Value=0.00193185138639
  Math Function : Math  Operator=pow  OutputSignalType=auto
  Math Function1 : Math  Operator=pow  OutputSignalType=auto
  Mux : Mux  Inputs=3
  One : Constant  Value=1
  Product : Product  Inputs=2  Multiplication=Element-wise(.*)  SaturateOnIntegerOverflow=on
  Product1 : Product  Inputs=**/  Multiplication=Element-wise(.*)  SaturateOnIntegerOverflow=on
  Product2 : Product  Inputs=*/  Multiplication=Element-wise(.*)  SaturateOnIntegerOverflow=on
  Product3 : Product  Inputs=2  Multiplication=Element-wise(.*)  SaturateOnIntegerOverflow=on
  Product4 : Product  Inputs=**/  Multiplication=Element-wise(.*)  SaturateOnIntegerOverflow=on
  Product5 : Product  Inputs=2  Multiplication=Element-wise(.*)  SaturateOnIntegerOverflow=on
  Sum : Sum  Inputs=|+-  SaturateOnIntegerOverflow=on
  Sum1 : Sum  Inputs=|+-  SaturateOnIntegerOverflow=on
  Sum2 : Sum  Inputs=|++  SaturateOnIntegerOverflow=on
  Terminator : Terminator
  eps^2 : Math  Operator=square  OutputSignalType=auto
  g(phi,h) : Fcn  Expr=u[1]-(3.0877e-6 - 0.0044e-6*u[2])*u[3]+0.072e-12*u[3]*u[3]
  sin(phi) : Trigonometry  Operator=sin  OutputSignalType=auto
  sin(phi)^2 : Math  Operator=square  OutputSignalType=auto
  sqrt : Math  Operator=sqrt  OutputSignalType=auto
  Rmeridian : Outport  Port=1
  Rnormal : Outport  Port=2
  Re : Outport  Port=3
  Gravity : Outport  Port=4
  wires:
  sqrt/1 -> Re/1
  Product5/1 -> sqrt/1
  First Eccentricity/1 -> eps^2/1
  eps^2/1 -> Sum/2, Product/1
  sin(phi)/1 -> sin(phi)^2/1
  sin(phi)^2/1 -> Product/2, Product3/2, Mux/2
  One/1 -> Sum1/1, Sum2/1, Sum/1
  Product/1 -> Sum1/2
  Sum1/1 -> Math Function/1, Math Function1/1
  3/2/1 -> Math Function/2
  1/2/1 -> Math Function1/2
  Equatorial Radius/1 -> Product1/1, Product2/1
  Sum/1 -> Product1/2
  Math Function/1 -> Product1/3
  Math Function1/1 -> Product2/2, Product4/3
  Product1/1 -> Rmeridian/1, Product5/1
  Product2/1 -> Rnormal/1, Product5/2
  Gravity formula const/1 -> Product3/1
  Product3/1 -> Sum2/2
  Gravity at Equator/1 -> Product4/1
  Sum2/1 -> Product4/2
  Product4/1 -> Mux/1
  Position/1 -> Demux2/1
  Demux2/1 -> sin(phi)/1
  Demux2/2 -> Terminator/1
  Mux/1 -> g(phi,h)/1
  g(phi,h)/1 -> Gravity/1
  Demux2/3 -> Mux/3

== system tp333079/Earth/WMM-2000 ==
  Position : Inport  Port=1  PortDimensions=[3 1]  SampleTime=-1  DataType=double
      settings: SignalType=auto
  DCM : Inport  Port=2  PortDimensions=[3 3]  SampleTime=-1  DataType=double
      settings: SignalType=auto
  Date : Constant  Value=simdate
  DayToYear : Gain  Gain=1/365  Multiplication=Element-wise(K.*u)  SaturateOnIntegerOverflow=on
  Demux : Demux  Outputs=3  BusSelectionMode=off
  Demux1 : Demux  Outputs=3  BusSelectionMode=off
  MonthToYear : Gain  Gain=1/12  Multiplication=Element-wise(K.*u)  SaturateOnIntegerOverflow=on
  Mux : Mux  Inputs=3
  Product : Product  Inputs=2  Multiplication=Matrix(*)  SaturateOnIntegerOverflow=on
  S-Function : S-Function  FunctionName=sfunwmm  Parameters=wmmfile  PortCounts=[]  SFunctionModules=''
  Sum : Sum  Inputs=+++  SaturateOnIntegerOverflow=on
  MagField : Outport  Port=1
  wires:
  S-Function/1 -> Product/2
  DCM/1 -> Product/1
  Date/1 -> Demux/1
  Demux/1 -> DayToYear/1
  DayToYear/1 -> Sum/1
  Demux/2 -> MonthToYear/1
  Demux/3 -> Sum/3
  MonthToYear/1 -> Sum/2
  Position/1 -> S-Function/1
  Sum/1 -> S-Function/2
  Product/1 -> Demux1/1
  Demux1/1 -> Mux/1
  Demux1/2 -> Mux/2
  Demux1/3 -> Mux/3
  Mux/1 -> MagField/1

== system tp333079/Equations of Motion/Body-Frame EOM ==
  Forces : Subsystem  SimViewingDevice=off  mask(Force equations){VelocitiesIni=VelocitiesIni}
      mask prompts: VelocitiesIni "Initial velocities:"
      mask help: 6-DOF rigid body force equations.
      settings: Permissions=ReadWrite  RTWFcnNameOpts=Auto  RTWFileNameOpts=Auto
      mask Help:
      | The block implements the 6-DOF rigid-body force equations.
      | <P><B>Inputs:</B>
      | <LI>Rates = the 3x1 vector of body angular rates</LI>
      | <LI>Accel = the 3x1 vector of linear body accelerations</LI>
      | <LI>Gravity = the gravitational acceleration at current location.
      | <LI>DCM = the 3x3 rotation matrix from navigation to body frame.
      | <LI>RST = the integrator reset flag (rising edge)</LI>
      | </P>
      | <P><B>Output:</B>
      | <LI>Velocities = the 3x1 vector of aircraft velocities in body axes</LI>
      | </P>
      | <P><B>Parameters:</B>
      | <LI>Initial velocities = the 3x1 vector of initial aircraft velocities</LI>
      | </P>
  Kinematics (Euler) : Subsystem  SimViewingDevice=off  mask(Kinematic Equations){EulerIni=EulerIni}
      mask prompts: EulerIni "Initial Euler angles:"
      mask help: 6-DOF rigid body kinematic equations, using Euler angles.
      settings: Permissions=ReadWrite  RTWFcnNameOpts=Auto  RTWFileNameOpts=Auto
      mask Help:
      | The block implements the 6-DOF rigid-body kinematic equations, using Euler angles.
      | <P><B>Inputs:</B>
      | <LI>Rates = the 3x1 vector of body angular rates</LI>
      | <LI>RST = the integrator reset flag (rising edge)</LI>
      | </P>
      | <P><B>Output:</B>
      | <LI>Euler = the 3x1 vector of Euler angles</LI>
      | </P>
      | <P><B>Parameters:</B>
      | <LI>Initial Euler angles = the 3x1 vector of initial body attitude</LI>
      | </P>
  Kinematics (Quaternions) : Subsystem  SimViewingDevice=off  mask(Kinematic Equations){QuaternionsIni=QuaternionsIni}
      mask prompts: QuaternionsIni "Initial quaternions:"
      mask help: 6-DOF rigid body kinematic equations, using Euler-Rodrigues quaternions.
      settings: Permissions=ReadWrite  RTWFcnNameOpts=Auto  RTWFileNameOpts=Auto
      mask Help:
      | The block implements the 6-DOF rigid-body kinematic equations, using Euler-Rodrigues quaternions.
      | <P><B>Inputs:</B>
      | <LI>Rates = the 3x1 vector of body angular rates</LI>
      | <LI>RST = the integrator reset flag (rising edge)</LI>
      | </P>
      | <P><B>Output:</B>
      | <LI>Quaternions = the 4x1 vector of body quaternions</LI>
      | </P>
      | <P><B>Parameters:</B>
      | <LI>Initial quaternions = the 4x1 vector of initial body quaternions</LI>
      | </P>
  Moments : Subsystem  SimViewingDevice=off  mask(Moment equations){RatesIni=RatesIni}
      mask prompts: RatesIni "Initial angular rates:"
      mask help: 6-DOF rigid body moment equations.
      settings: Permissions=ReadWrite  RTWFcnNameOpts=Auto  RTWFileNameOpts=Auto
      mask Help:
      | The block implements the 6-DOF rigid-body moment equations.
      | <P><B>Inputs:</B>
      | <LI>Inertia = the 10x1 vector of inertia coefficients</LI>
      | <LI>Moments = the 3x1 vector of airframe moments</LI>
      | <LI>RST = the integrator reset flag (rising edge)</LI>
      | </P>
      | <P><B>Output:</B>
      | <LI>Angular Rates = the 3x1 vector of body angular rates</LI>
      | <LI>Angular Acc = the 3x1 vector of body angular accelerations.
      | </P>
      | <P><B>Parameters:</B>
      | <LI>Initial rates = the 3x1 vector of initial angular rates</LI>
      | </P>
  Navigation : Subsystem  SimViewingDevice=off  mask(Navigation equations){PositionIni=PositionIni}
      mask prompts: PositionIni "Initial position:"
      mask help: 6-DOF rigid body navigation equations.
      settings: Permissions=ReadWrite  RTWFcnNameOpts=Auto  RTWFileNameOpts=Auto
      mask Help:
      | The block implements the inertial navigation equations.
      | <P><B>Inputs:</B>
      | <LI>Velocities = the 3x1 vector of aircraft velocities in body axes</LI>
      | <LI>DCM = the 3x3 frame transformation from navigation frame to body frame</LI>
      | <LI>Rmeridian = the Earth meridian radius, in m</LI>
      | <LI>Rnormal = the Earth normal radius, in m</LI>
      | <LI>AConGnd = the aircraft-on-ground flag</LI>
      | <LI>RST = the integrator reset flag (rising edge)</LI>
      | </P>
      | <P><B>Output:</B>
      | <LI>Position = the 3x1 vector of aircraft location [Latitude Longitude Altitude] in [rad rad m]</LI>
      | <LI>Gndspd = the 3x1 vector of aircraft velocities in navigation frame [North East Down] in m/s</LI>
      | </P>
      | <P><B>Parameters:</B>
      | <LI>Initial position = the 3x1 vector of initial aircraft position</LI>
      | </P>

== system tp333079/Equations of Motion/Geodetic-Frame EOM ==
  Angular Rate : Subsystem  SimViewingDevice=off  mask(Angular rate equations){RatesIni=}
      mask prompts: RatesIni "Initial angular rates:"
      mask help: The angular rate equations in body frame which take the Earth rotation rate into account.
      settings: Permissions=ReadWrite  RTWFcnNameOpts=Auto  RTWFileNameOpts=Auto
      mask Help:
      | The block implements the body angular rate equations by integrating the moments applied to the airframe and adding the Earth rotation rate components in body axes.
      | <P><B>Inputs:</B>
      | <LI>Inertia = the 10x1 vector of inertia coefficients</LI>
      | <LI>Moments = the 3x1 vector of airframe moments</LI>
      | <LI>Pos = the 3x1 vector of aircraft geodetic position [Lat Lon Alt]
      | <LI>dPosdt = the 3x1 vector of aircraft position derivatives
      | <LI>DCM = the 3x3 navigation-to-body frame transformation matrix
      | <LI>RST = the integrator reset flag (rising edge)</LI>
      | </P>
      | <P><B>Output:</B>
      | <LI>Angular Rate = the 3x1 vector of body angular rates</LI>
      | <LI>Angular Acc = the 3x1 vector of body angular accelerations.
      | </P>
      | <P><B>Parameters:</B>
      | <LI>Initial rates = the 3x1 vector of initial angular rates</LI>
      | </P>
  Attitude (Euler) : aerosimlib/Equations of Motion/Body-Frame EOM/Kinematics (Euler)  EulerIni=EulerIni
  Attitude (Quaternions) : aerosimlib/Equations of Motion/Body-Frame EOM/Kinematics (Quaternions)  QuaternionsIni=QuaternionsIni
  Position : Subsystem  SimViewingDevice=off  mask(Position equations){PositionIni=PositionIni}
      mask prompts: PositionIni "Initial position:"
      mask help: Position equations in geodetic frame. Assumes WGS-84 Earth geoid model.
      settings: Permissions=ReadWrite  RTWFcnNameOpts=Auto  RTWFileNameOpts=Auto
      mask Help:
      | The block implements the inertial position equations in geodetic frame (North-East-Down).
      | <P><B>Inputs:</B>
      | <LI>Vel NED = the 3x1 vector of aircraft velocities in geodetic frame</LI>
      | <LI>Rmeridian = the Earth meridian radius, in m</LI>
      | <LI>Rnormal = the Earth normal radius, in m</LI>
      | <LI>AConGnd = the aircraft-on-ground flag</LI>
      | <LI>RST = the integrator reset flag (rising edge)</LI>
      | </P>
      | <P><B>Output:</B>
      | <LI>Position = the 3x1 vector of aircraft location [Latitude Longitude Altitude] in [rad rad m]</LI>
      | <LI>dPosdt = the 3x1 vector of aircraft position derivatives in m/s</LI>
      | </P>
      | <P><B>Parameters:</B>
      | <LI>Initial position = the 3x1 vector of initial aircraft position</LI>
      | </P>
  Velocity : Subsystem  SimViewingDevice=off  mask(Velocity Equations){VelocitiesIni=VelocitiesIni}
      mask prompts: VelocitiesIni "Initial velocities:"
      mask help: The velocity equations in geodetic frame.
      settings: Permissions=ReadWrite  RTWFcnNameOpts=Auto  RTWFileNameOpts=Auto
      mask Help:
      | The block implements the velocity equations in geodetic frame (North-East-Down).
      | <P><B>Inputs:</B>
      | <LI>Pos = the 3x1 vector of aircraft position [Lat Lon Alt];
      | <LI>dPosdt = the 3x1 vector of aircraft position derivatives;
      | <LI>Accel = the 3x1 vector of linear body accelerations</LI>
      | <LI>DCM = the 3x3 rotation matrix from navigation to body frame.
      | <LI>Gravity = the gravitational acceleration at current location.
      | <LI>RST = the integrator reset flag (rising edge)</LI>
      | </P>
      | <P><B>Output:</B>
      | <LI>Velocity NED = the 3x1 vector of aircraft velocities in geodetic frame</LI>
      | </P>
      | <P><B>Parameters:</B>
      | <LI>Initial velocities = the 3x1 vector of initial aircraft velocities in geodetic frame</LI>
      | </P>

== system tp333079/Equations of Motion/Total Acceleration ==
  note: Sources
  Faero : Inport  Port=1  PortDimensions=[3 1]  SampleTime=-1  DataType=auto
      settings: SignalType=auto
  Fprop : Inport  Port=2  PortDimensions=[3 1]  SampleTime=-1  DataType=auto
      settings: SignalType=auto
  Mass : Inport  Port=3  PortDimensions=1  SampleTime=-1  DataType=auto
      settings: SignalType=auto
  F/m : Product  Inputs=*/  Multiplication=Element-wise(.*)  SaturateOnIntegerOverflow=on
  Sum1 : Sum  Inputs=++  SaturateOnIntegerOverflow=on
  Acc : Outport  Port=1
  wires:
  F/m/1 -> Acc/1
  Mass/1 -> F/m/2
  Sum1/1 -> F/m/1
  Fprop/1 -> Sum1/2
  Faero/1 -> Sum1/1

== system tp333079/Equations of Motion/Total Moment ==
  note: Sources
  note: Moments at CG created by aero and propulsion forces
  note: Total moments at CG location
  Faero : Inport  Port=1  PortDimensions=[3 1]  SampleTime=-1  DataType=auto
      settings: SignalType=auto
  Maero : Inport  Port=2  PortDimensions=[3 1]  SampleTime=-1  DataType=auto
      settings: SignalType=auto
  Fprop : Inport  Port=3  PortDimensions=[3 1]  SampleTime=-1  DataType=auto
      settings: SignalType=auto
  Mprop : Inport  Port=4  PortDimensions=[3 1]  SampleTime=-1  DataType=auto
      settings: SignalType=auto
  CGpos : Inport  Port=5  PortDimensions=[3 1]  SampleTime=-1  DataType=auto
      settings: SignalType=auto
  Aero Moment : Subsystem  SimViewingDevice=off
      settings: Permissions=ReadWrite  RTWFcnNameOpts=Auto  RTWFileNameOpts=Auto
  Propulsion Moment : Subsystem  SimViewingDevice=off
      settings: Permissions=ReadWrite  RTWFcnNameOpts=Auto  RTWFileNameOpts=Auto
  Sum : Sum  Inputs=|+-  SaturateOnIntegerOverflow=on
  Sum1 : Sum  Inputs=++++  SaturateOnIntegerOverflow=on
  Sum2 : Sum  Inputs=|+-  SaturateOnIntegerOverflow=on
  r_aero : Constant  Value=raero
  r_prop : Constant  Value=rprop
  Mcg : Outport  Port=1
  wires:
  Propulsion Moment/1(ProdVec) -> Sum1/4
  Maero/1 -> Sum1/1
  Fprop/1 -> Propulsion Moment/2(Vec2)
  Mprop/1 -> Sum1/3
  Aero Moment/1(ProdVec) -> Sum1/2
  Sum1/1 -> Mcg/1
  Faero/1 -> Aero Moment/2(Vec2)
  r_aero/1 -> Sum2/1
  r_prop/1 -> Sum/1
  CGpos/1 -> Sum2/2, Sum/2
  Sum/1 -> Propulsion Moment/1(Vec1)
  Sum2/1 -> Aero Moment/1(Vec1)

== system tp333079/FlightGear-Compatible/Aerodynamics ==
  Coefficient : Subsystem  BlockChoice=Value  SimViewingDevice=off
      settings: TemplateBlock=self  MemberBlocks=Table,Value,Vector  Permissions=ReadWrite  RTWFcnNameOpts=Auto  RTWFileNameOpts=Auto
  Table : Subsystem  SimViewingDevice=off  mask(Aerodynamic coefficient: Table){Table=0}
      mask prompts: Table "Coefficient:"
      mask help: The block implements a 2-D look-up table aerodynamic coefficient.
      settings: Permissions=ReadWrite  RTWFcnNameOpts=Auto  RTWFileNameOpts=Auto
      mask Help:
      | The block implements a 2-D look-up table aerodynamic coefficient.
      | <P><B>Inputs:</B>
      | <LI>RowParam = the row argument for the look-up table</LI>
      | <LI>ColParam = the column argument for the look-up table</LI>
      | </P>
      | <P><B>Outputs:</B>
      | <LI>Coeff = the aerodynamic coefficient</LI>
      | </P>
      | <P><B>Parameters:</B>
      | <LI>Coefficient = the Matlab structure for a table-coefficient.</LI>
      | </P>
  Value : Subsystem  SimViewingDevice=off  mask(Aerodynamic coefficient: Value){Value=0}
      mask prompts: Value "Coefficient:"
      mask help: The block implements a scalar aerodynamic coefficient.
      settings: Permissions=ReadWrite  RTWFcnNameOpts=Auto  RTWFileNameOpts=Auto
      mask Help:
      | The block implements a scalar aerodynamic coefficient.
      | <P><B>Inputs:</B>
      | <LI>RowParam = the input argument</LI>
      | </P>
      | <P><B>Outputs:</B>
      | <LI>Coeff = the aerodynamic coefficient</LI>
      | </P>
      | <P><B>Parameters:</B>
      | <LI>Coefficient = the Matlab value-coefficient structure</LI>
      | </P>
  Vector : Subsystem  SimViewingDevice=off  mask(Aerodynamic coefficient: Vector){Vector=0}
      mask prompts: Vector "Coefficient:"
      mask help: The block implements a vector (1-D look-up-table) aerodynamic coefficient.
      settings: Permissions=ReadWrite  RTWFcnNameOpts=Auto  RTWFileNameOpts=Auto
      mask Help:
      | The block implements a vector (1-D look-up-table) aerodynamic coefficient.
      | <P><B>Inputs:</B>
      | <LI>RowParam = the input argument</LI>
      | </P>
      | <P><B>Outputs:</B>
      | <LI>Coeff = the aerodynamic coefficient</LI>
      | </P>
      | <P><B>Parameters:</B>
      | <LI>Coefficient = the Matlab structure of a vector coefficient</LI>
      | </P>
